simulink library "NUbotsUDP"  (R2019b)
settings: Solver=VariableStepAuto  StartTime=0.0  StopTime=10.0  RelTol=1e-3
libraries: instrumentlib x2
settings Model: Creator=cameron  LastModifiedBy=cameron

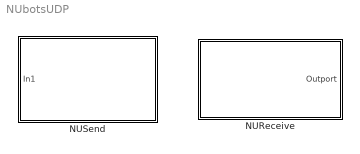
== system NUbotsUDP ==
  NUReceive : Subsystem  mask(NUReceive){LocalPort=5002, RemotePort=5001}
      mask help: Revices Data from Remote Port to Local Port
      mask init:
      | set_param([gcb '/UDP Receive'], 'LocalPort', get_param(gcb,'LocalPort'));
      | set_param([gcb '/UDP Receive'], 'Port', get_param(gcb,'RemotePort'));
      | %TODO Sample Time
      mask Display:
      | disp(['LocalPort: ' get_param(gcb,'LocalPort') '\n\n']);
      | disp(['RemotePort: ' get_param(gcb,'RemotePort')]);
  NUSend : Subsystem  mask(NUSend){LocalPort=5001, RemotePort=5002}
      mask help:
      | Sends data to Remote Port from Local Port.
      |
      | The input should be a struct of integers.
      mask init:
      | set_param([gcb '/UDP Send'], 'LocalPort', get_param(gcb,'LocalPort'));
      | set_param([gcb '/UDP Send'], 'Port', get_param(gcb,'RemotePort'));
      mask Display:
      | disp(['LocalPort: ' get_param(gcb,'LocalPort') '\n\n']);
      | disp(['RemotePort: ' get_param(gcb,'RemotePort')]);

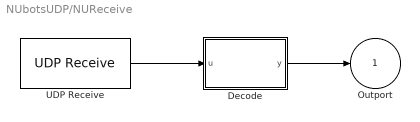
== system NUbotsUDP/NUReceive ==
  "Decode " : MATLAB Function  TreatAsAtomicUnit=on
  UDP Receive : instrumentlib/UDP Receive  Priority=3  Host=localhost  Port=5001  LocalPort=5002  EnablePortSharing=off  GetLatestData=off  DataSize="[145    1]"  DataType=uint8  ASCIIFormatting=%d  Terminator=LF  ByteOrder=BigEndian  EnableBlockingMode=on  Timeout=5  SampleTime=0.1  LocalAddress=0.0.0.0
      settings: SourceProductName=Instrument Control Toolbox
  Outport : Outport  OutDataTypeStr=double  PortDimensions=16
  wires:
  UDP Receive/1 -> "Decode "/1(u)
  "Decode "/1(y) -> Outport/1

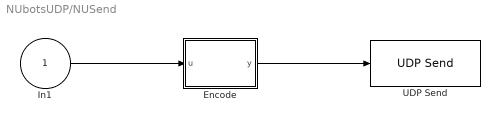
== system NUbotsUDP/NUSend ==
  In1 : Inport  OutDataTypeStr=double  PortDimensions=16
  Encode : MATLAB Function  TreatAsAtomicUnit=on
  UDP Send : instrumentlib/UDP Send  Priority=2  Host=localhost  Port=5002  LocalPort=5001  EnablePortSharing=off  ByteOrder=BigEndian  OutputDatagramPacketSize=256  EnableBlockingMode=off  LocalAddress=0.0.0.0
      settings: SourceProductName=Instrument Control Toolbox
  wires:
  In1/1 -> Encode/1(u)
  Encode/1(y) -> UDP Send/1

== matlab function NUbotsUDP/NUReceive/Decode  ==
  data: u input; y output
function y = fcn(u)
y = zeros(16,1,'double');
coder.extrinsic('ProtobufDecode'); 
y = ProtobufDecode(u);

== matlab function NUbotsUDP/NUSend/Encode ==
  data: u input; y output
function y = fcn(u)
coder.extrinsic('ProtobufEncode');
t = ProtobufEncode(u);
s = size(t);
y = zeros(s(1),'uint8');
